simulink model "main_test"  (R2022a)
settings: Solver=VariableStepAuto  StartTime=0.0  StopTime=6  RelTol=1e-3
undefined symbols (not defined in the file): Acid, Lead
libraries: spsSeriesRLCBranchLib x3, spsDiodeLib x2, spsBatteryLib x1, spsCurrentMeasurementLib x1, spsMosfetLib x1, spsPVArrayLib x1, simulink x1, spspowerguiLib x1
settings Model: Creator=asher  LastModifiedBy=asher

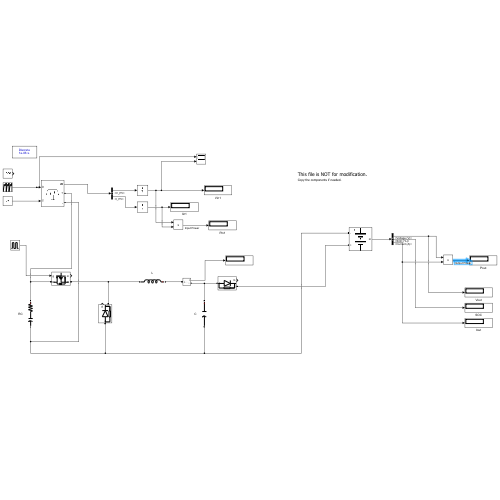
[thumbnail: Simulink's stored preview of the top-level diagram]
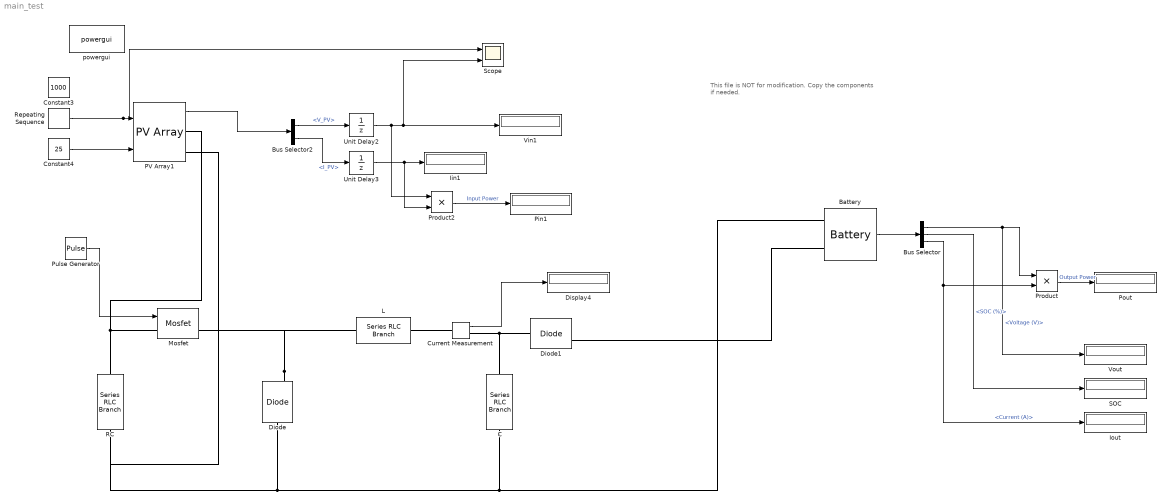
== system main_test ==
  note: This file is NOT for modification.
      | Copy the components if needed.
  Battery : spsBatteryLib/Battery  BatType=Lead-Acid  ShowTempParam=off  ThermalPreset=no  ShowAgeParam=off  NomV=15  NomQ=100  SOC=30  Batt_Tr=10  PresetModel=on  MaxQ=104.1667  MinV=11.25  FullV=16.3322  Dis_rate=20  R=0.0015  Normal_OP=31.0278  expZone="[15.2714     0.333333]"  current=[6.5 13 32.5]  Units=Time  Tci=20  NomT=20  T2=-30  MaxQ2=4.8  FullV2=7.1  Normal_OP2=5.655  expZone2="[6.58           1]"  Rca=0.6  ti=2000  Dp=0  Neq0=0  Tsim=1e6  Ta1=25  Qeol=5.4*0.9  Reol=0.013333*1.2  Char_age=[2.3478, 3]  Dis_age=[2.3478, 10]  N1=1500  N2=10500  N3=1000  N4=1400  Ta2=45  N5=950
  Bus Selector : BusSelector  OutputSignals=Voltage (V),SOC (%),Current (A)
  Bus Selector2 : BusSelector  OutputSignals=V_PV,I_PV
  C : spsSeriesRLCBranchLib/Series RLC Branch  LConnTagsString=__new0  RConnTagsString=__new0  BranchType=C  Resistance=1  Inductance=1e-3  SetiL0=off  InitialCurrent=0  Capacitance=933e-6  Setx0=off  InitialVoltage=0  Measurements=None
  Constant3 : Constant  Value=1000
  Constant4 : Constant  Value=25
  Current Measurement : spsCurrentMeasurementLib/Current Measurement  PhasorSimulation=off  OutputType=Complex  PSBequivalent=0
  Diode : spsDiodeLib/Diode  Ron=0.001  Lon=0  Vf=0.8  IC=0  UseSnubber=0  Rs=500  Cs=250e-9  Measurements=on
  Diode1 : spsDiodeLib/Diode  Ron=0.001  Lon=0  Vf=0.8  IC=0  UseSnubber=0  Rs=500  Cs=250e-9  Measurements=on
  Display4 : Display
  Iin1 : Display
  Iout : Display
  L : spsSeriesRLCBranchLib/Series RLC Branch  LConnTagsString=__new0  RConnTagsString=__new0  BranchType=L  Resistance=1  Inductance=9.949e-6  SetiL0=off  InitialCurrent=0  Capacitance=1e-6  Setx0=off  InitialVoltage=0  Measurements=None
  Mosfet : spsMosfetLib/Mosfet  Ron=0.1  Lon=0  Rd=0.01  Vfd=0  IC=0  Rs=1e5  Cs=inf  Measurements=on
  PV Array1 : spsPVArrayLib/PV Array  Npar=1  Nser=1  PlotType=array @ 25 deg.C & specified irradiances  S_vec="[ 1000  500  100 ]"  Temp_C_vec="[ 45 25  ]"  ModuleName=User-defined  PlotWhenSelected=off  Pm=213.15  Ncell=60  Voc=36.3  Isc=7.84  Vm=29  Im=7.35  beta_Voc_pc=-0.36099  alpha_Isc_pc=0.102  beta_Voc=-0.13104  alpha_Isc=0.0079968  IL=7.8654  I0=2.9273e-10  nI=0.98119  Rsh=313.0553  Rs=0.39381  RobustModel=off  RobustCellTemperature=313.3991  BAL=on  Tc=1e-6  Tfilter=5e-5
  Pin1 : Display
  Pout : Display
  Product : Product
  Product2 : Product
  Pulse Generator : DiscretePulseGenerator  PulseType=Time based  Period=2e-5  PulseWidth=53.57
  RC : spsSeriesRLCBranchLib/Series RLC Branch  LConnTagsString=__new0  RConnTagsString=__new0  BranchType=RC  Resistance=0.0001  Inductance=1e-3  SetiL0=off  InitialCurrent=0  Capacitance=0.001  Setx0=off  InitialVoltage=0  Measurements=None
  Repeating Sequence : simulink/Sources/Repeating Sequence  rep_seq_t=[0 2 4 6]  rep_seq_y=[0 1000 800 1200]
  SOC : Display
  Scope : Scope  NumInputPorts=2
  Unit Delay2 : UnitDelay  SampleTime=-1  HasFrameUpgradeWarning=on
  Unit Delay3 : UnitDelay  SampleTime=-1  HasFrameUpgradeWarning=on
  Vin1 : Display
  Vout : Display
  powergui : spspowerguiLib/powergui  Priority=1  SimulationMode=Discrete  SampleTime=1e-6  frequency=60  Iterations=50  frequencyindice=0  Pbase=100e6  ErrMax=1e-4  UnitsV=kV  UnitsW=MW  buscounter=0  FunctionMessages=off  echomessages=off  EnableUseOfTLC=off  CurrentSourceSwitches=off  DisableSnubberDevices=off  DisableRonSwitches=off  DisableVfSwitches=off  DisplayEquations=off  AutomaticDiscreteSolvers=off  SolverType=Tustin/Backward Euler (TBE)  Interpol=off  ExternalGateDelay=off  methode=off  Ts=100  x0status=blocks  SPID=on  SwTol=0  HookPort=off  NonlinearTolerance=1e-4  nMaxIteration=100  ContinueOnMaxIteration=off  RestoreLinks=warning  ResistiveCurrentMeasurement=off  Frange=[0:2:500]  Ylog=off  Xlog=on  ShowGrid=off  save=off  variable=ZData  structure=0  ZoomFFT=off  StartTime=0.0  cycles=1  DisplayStyle=1  fundamental=60  FreqAxis=off  MaxFrequency=1000  frequencyindicesteady=1  RmsSteady=1  display=off
  wires:
  Product2/1 -> Pin1/1  "Input Power"
  Unit Delay3/1 -> Product2/2, Iin1/1
  Unit Delay2/1 -> Product2/1, Scope/2, Vin1/1
  Bus Selector2/1 -> Unit Delay2/1  "<V_PV>"
  Bus Selector2/2 -> Unit Delay3/1  "<I_PV>"
  Constant4/1 -> PV Array1/2
  PV Array1/1 -> Bus Selector2/1
  Current Measurement/1 -> Display4/1
  Pulse Generator/1 -> Mosfet/1
  Product/1 -> Pout/1  "Output Power"
  Bus Selector/2 -> SOC/1  "<SOC (%)>"
  Battery/1 -> Bus Selector/1
  Bus Selector/3 -> Product/2, Iout/1  "<Current (A)>"
  Bus Selector/1 -> Product/1, Vout/1  "<Voltage (V)>"
  Repeating Sequence/1 -> Scope/1, PV Array1/1
  connections:
  RC/LConn1 -- PV Array1/RConn1 -- Mosfet/LConn1
  Diode/RConn1 -- Mosfet/RConn1 -- L/RConn1
  PV Array1/RConn2 -- RC/RConn1 -- Diode/LConn1 -- C/RConn1 -- Battery/LConn2
  Diode1/LConn1 -- Current Measurement/RConn1 -- C/LConn1
  Current Measurement/LConn1 -- L/LConn1
  Battery/LConn1 -- Diode1/RConn1
